simulink model "sim"  (R2021a)
settings: Solver=VariableStepAuto  StartTime=0.0  StopTime=150  RelTol=1e-3
settings Model: Creator=Abbas  LastModifiedBy=Abbas

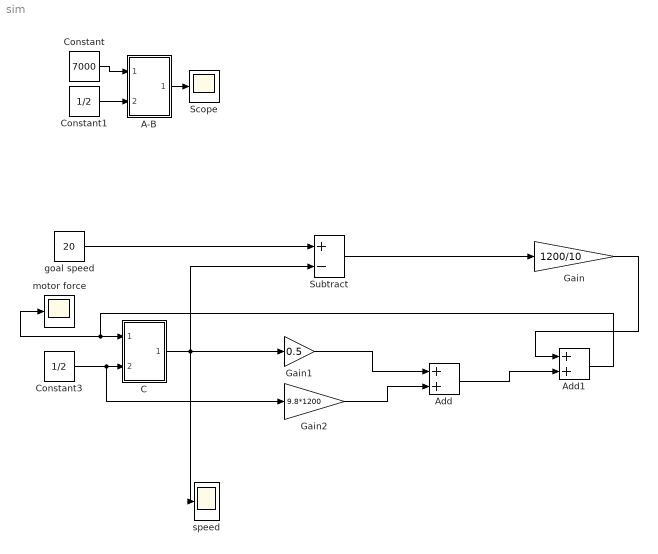
== system sim ==
  A-B : Subsystem
  Add : Sum
  Add1 : Sum
  C : Subsystem
  Constant : Constant  Value=7000
  Constant1 : Constant  Value=1/2
  Constant3 : Constant  Value=1/2
  Gain : Gain  Gain=1200/10
  Gain1 : Gain  Gain=0.5
  Gain2 : Gain  Gain=9.8*1200
  Scope : Scope
  Subtract : Sum  Inputs=+-
  goal speed : Constant  Value=20
  motor force : Scope
  speed : Scope
  wires:
  Constant/1 -> A-B/1(In1)
  Constant1/1 -> A-B/2(In3)
  A-B/1(Out1) -> Scope/1
  C/1(Out1) -> Gain1/1, Subtract/2, speed/1
  Constant3/1 -> Gain2/1, C/2(In3)
  Gain/1 -> Add1/1
  goal speed/1 -> Subtract/1
  Subtract/1 -> Gain/1
  Gain1/1 -> Add/1
  Gain2/1 -> Add/2
  Add/1 -> Add1/2
  Add1/1 -> C/1(In1), motor force/1

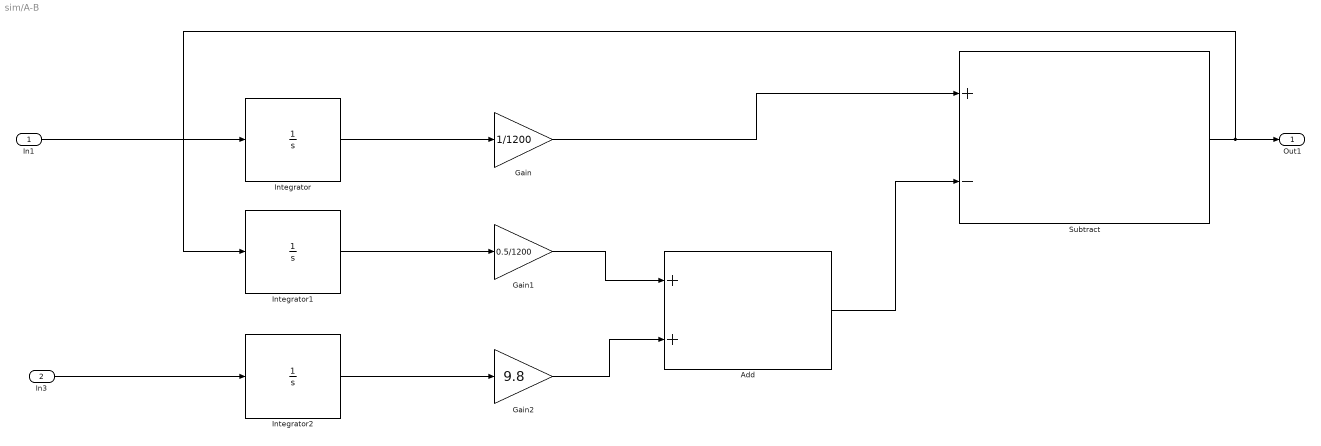
== system sim/A-B ==
  In1 : Inport
  In3 : Inport  Port=2
  Add : Sum
  Gain : Gain  Gain=1/1200
  Gain1 : Gain  Gain=0.5/1200
  Gain2 : Gain  Gain=9.8
  Integrator : Integrator
  Integrator1 : Integrator
  Integrator2 : Integrator
  Subtract : Sum  Inputs=+-
  Out1 : Outport
  wires:
  Integrator1/1 -> Gain1/1
  Integrator/1 -> Gain/1
  Integrator2/1 -> Gain2/1
  Gain1/1 -> Add/1
  Gain2/1 -> Add/2
  Add/1 -> Subtract/2
  In1/1 -> Integrator/1
  Gain/1 -> Subtract/1
  Subtract/1 -> Integrator1/1, Out1/1
  In3/1 -> Integrator2/1

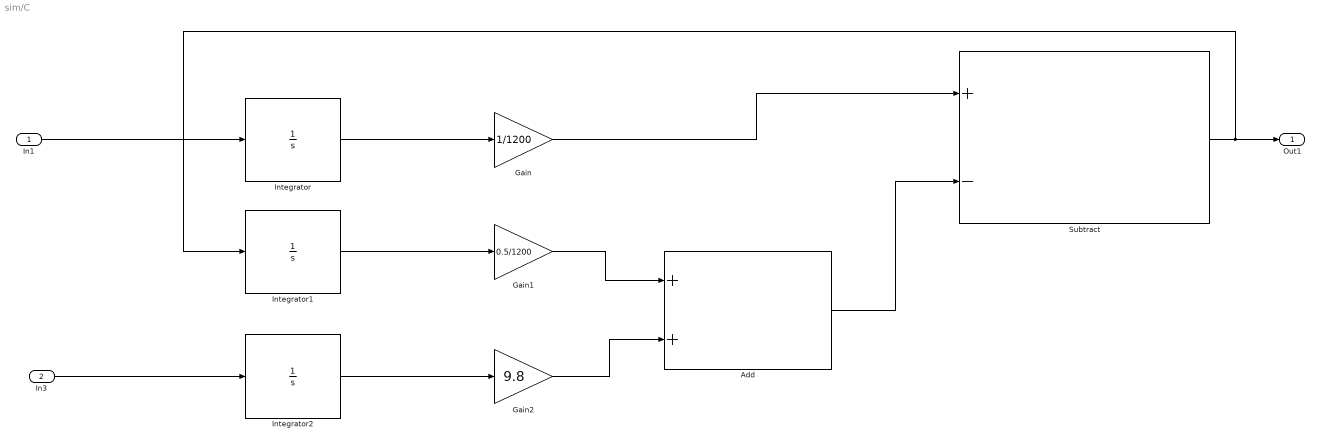
== system sim/C ==
  In1 : Inport
  In3 : Inport  Port=2
  Add : Sum
  Gain : Gain  Gain=1/1200
  Gain1 : Gain  Gain=0.5/1200
  Gain2 : Gain  Gain=9.8
  Integrator : Integrator
  Integrator1 : Integrator
  Integrator2 : Integrator
  Subtract : Sum  Inputs=+-
  Out1 : Outport
  wires:
  Integrator1/1 -> Gain1/1
  Integrator/1 -> Gain/1
  Integrator2/1 -> Gain2/1
  Gain1/1 -> Add/1
  Gain2/1 -> Add/2
  Add/1 -> Subtract/2
  In1/1 -> Integrator/1
  Gain/1 -> Subtract/1
  Subtract/1 -> Integrator1/1, Out1/1
  In3/1 -> Integrator2/1
